simulink model "delay_on_off_prove"  (R2014b)
settings: Solver=FixedStepDiscrete  StartTime=0.0  StopTime=10.0  FixedStep=0.01  RelTol=1e-3
undefined symbols (not defined in the file): sldvsubsys
libraries: sldvlib x24
settings Model: ModifiedByFormat=Natasha  Creator=Natasha  LastModifiedBy=Natasha
settings DebuggingCC: UnderspecifiedInitializationDetection=Classic  MergeDetectMultiDrivingBlocksExec=none
settings ConfigComp: Description=Design Verifier Custom Configuration Component  DVMaxProcessTime=3600  DVMaxTestCaseSteps=500  DVTestSuiteOptimization=CombinedObjectives (Nonlinear Extended)  DVDetectActiveLogic=on

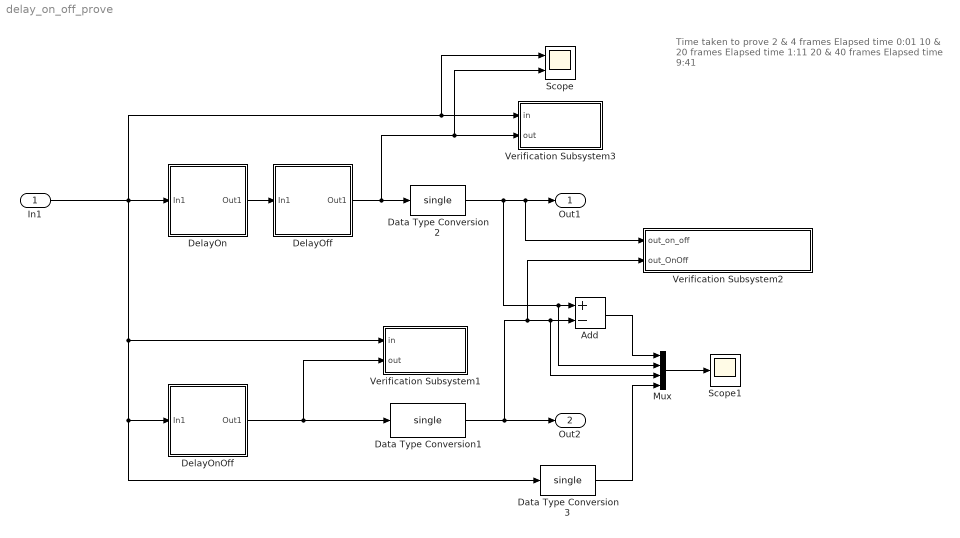
== system delay_on_off_prove ==
  note: Time taken to prove
      |
      | 2 & 4 frames Elapsed time 0:01
      | 10 & 20 frames Elapsed time 1:11
      | 20 & 40 frames Elapsed time 9:41
  In1 : Inport
  Add : Sum  Inputs=+-
  Data Type Conversion1 : DataTypeConversion  OutDataTypeStr=single
  Data Type Conversion2 : DataTypeConversion  OutDataTypeStr=single
  Data Type Conversion3 : DataTypeConversion  OutDataTypeStr=single
  DelayOff : Subsystem
  DelayOn : Subsystem
  DelayOnOff : Subsystem
  Mux : Mux
  Scope : Scope  NumInputPorts=2
      settings: YMin=-5~-5  YMax=5~5
  Scope1 : Scope
  Verification Subsystem1 : Subsystem  Tag=VerificationSubsystem  DisableCoverage=on  LoadFcn=sldvsubsys('check')  TreatAsAtomicUnit=on  SimViewingDevice=on  mask(VerificationSubsystem){}
      mask init:
      | sldvsubsys('maskInit');
      settings: CopyFcn=sldvsubsys('copy');  OpenFcn=open_system(gcb,'force');
      settings: PreSaveFcn=|
      | set_param(gcb,'SimViewingDevice','on');
      | sldvsubsys('check');
      mask Help: helpview(fullfile(docroot,'toolbox','sldv','sldv.map'),'verificationsubsystem')
      mask Display: image(imread('sldvicon_versubsys.png','BackGroundColor',[1 1 1]),'center');
  Verification Subsystem2 : Subsystem  Tag=VerificationSubsystem  DisableCoverage=on  LoadFcn=sldvsubsys('check')  TreatAsAtomicUnit=on  SimViewingDevice=on  mask(VerificationSubsystem){}
      mask init:
      | sldvsubsys('maskInit');
      settings: CopyFcn=sldvsubsys('copy');  OpenFcn=open_system(gcb,'force');
      settings: PreSaveFcn=|
      | set_param(gcb,'SimViewingDevice','on');
      | sldvsubsys('check');
      mask Help: helpview(fullfile(docroot,'toolbox','sldv','sldv.map'),'verificationsubsystem')
      mask Display: image(imread('sldvicon_versubsys.png','BackGroundColor',[1 1 1]),'center');
  Verification Subsystem3 : Subsystem  Tag=VerificationSubsystem  DisableCoverage=on  LoadFcn=sldvsubsys('check')  TreatAsAtomicUnit=on  SimViewingDevice=on  mask(VerificationSubsystem){}
      mask init:
      | sldvsubsys('maskInit');
      settings: CopyFcn=sldvsubsys('copy');  OpenFcn=open_system(gcb,'force');
      settings: PreSaveFcn=|
      | set_param(gcb,'SimViewingDevice','on');
      | sldvsubsys('check');
      mask Help: helpview(fullfile(docroot,'toolbox','sldv','sldv.map'),'verificationsubsystem')
      mask Display: image(imread('sldvicon_versubsys.png','BackGroundColor',[1 1 1]),'center');
  Out1 : Outport
  Out2 : Outport  Port=2
  wires:
  DelayOn/1(Out1) -> DelayOff/1(In1)
  DelayOff/1(Out1) -> Data Type Conversion2/1, Verification Subsystem3/2(out), Scope/2
  DelayOnOff/1(Out1) -> Verification Subsystem1/2(out), Data Type Conversion1/1
  Add/1 -> Mux/1
  Data Type Conversion1/1 -> Verification Subsystem2/2(out_OnOff), Mux/3, Add/2, Out2/1
  Data Type Conversion2/1 -> Mux/2, Add/1, Verification Subsystem2/1(out_on_off), Out1/1
  Mux/1 -> Scope1/1
  In1/1 -> Verification Subsystem3/1(in), Scope/1, Verification Subsystem1/1(in), Data Type Conversion3/1, DelayOnOff/1(In1), DelayOn/1(In1)
  Data Type Conversion3/1 -> Mux/4

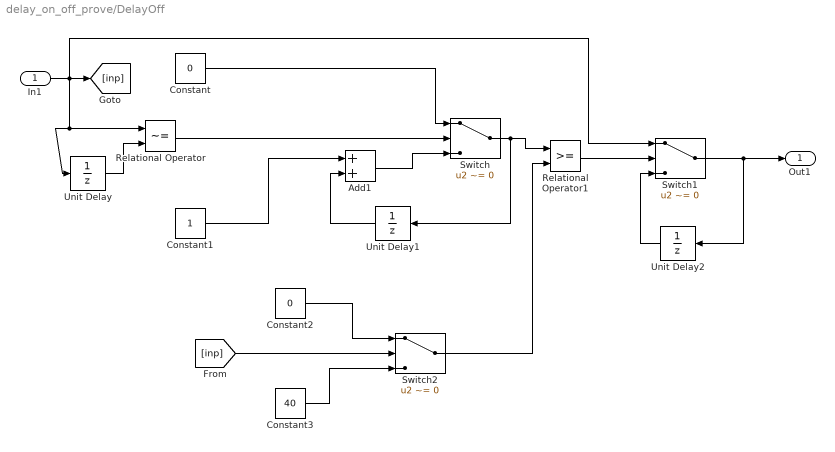
== system delay_on_off_prove/DelayOff ==
  In1 : Inport
  Add1 : Sum
  Constant : Constant  Value=0
  Constant1 : Constant
  Constant2 : Constant  Value=0
  Constant3 : Constant  Value=40
  Relational Operator : RelationalOperator  Operator=~=  OutDataTypeStr=boolean
  Relational Operator1 : RelationalOperator  OutDataTypeStr=boolean
  Switch : Switch  Criteria=u2 ~= 0
  Switch1 : Switch  Criteria=u2 ~= 0
  Switch2 : Switch  Criteria=u2 ~= 0
  Unit Delay : UnitDelay  SampleTime=-1
  Unit Delay1 : UnitDelay  SampleTime=-1
  Unit Delay2 : UnitDelay  SampleTime=-1
  Out1 : Outport
  wires:
  In1/1 -> [inp], Relational Operator/1, Unit Delay/1, Switch1/1
  [inp] -> Switch2/2
  Add1/1 -> Switch/3
  Switch2/1 -> Relational Operator1/2
  Constant3/1 -> Switch2/3
  Switch/1 -> Relational Operator1/1, Unit Delay1/1
  Relational Operator1/1 -> Switch1/2
  Unit Delay2/1 -> Switch1/3
  Switch1/1 -> Unit Delay2/1, Out1/1
  Unit Delay/1 -> Relational Operator/2
  Constant/1 -> Switch/1
  Relational Operator/1 -> Switch/2
  Constant1/1 -> Add1/1
  Constant2/1 -> Switch2/1
  Unit Delay1/1 -> Add1/2

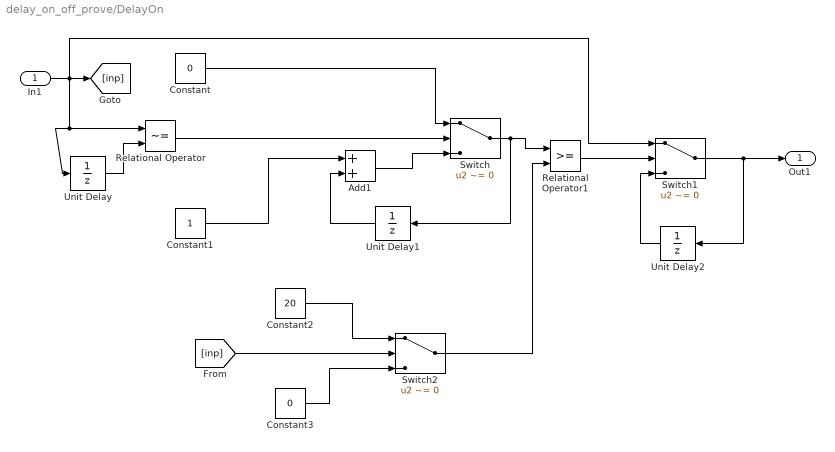
== system delay_on_off_prove/DelayOn ==
  In1 : Inport
  Add1 : Sum
  Constant : Constant  Value=0
  Constant1 : Constant
  Constant2 : Constant  Value=20
  Constant3 : Constant  Value=0
  Relational Operator : RelationalOperator  Operator=~=  OutDataTypeStr=boolean
  Relational Operator1 : RelationalOperator  OutDataTypeStr=boolean
  Switch : Switch  Criteria=u2 ~= 0
  Switch1 : Switch  Criteria=u2 ~= 0
  Switch2 : Switch  Criteria=u2 ~= 0
  Unit Delay : UnitDelay  SampleTime=-1
  Unit Delay1 : UnitDelay  SampleTime=-1
  Unit Delay2 : UnitDelay  SampleTime=-1
  Out1 : Outport
  wires:
  Unit Delay1/1 -> Add1/2
  Constant2/1 -> Switch2/1
  Constant1/1 -> Add1/1
  Relational Operator/1 -> Switch/2
  Constant/1 -> Switch/1
  Unit Delay/1 -> Relational Operator/2
  Switch1/1 -> Out1/1, Unit Delay2/1
  Unit Delay2/1 -> Switch1/3
  Relational Operator1/1 -> Switch1/2
  Switch/1 -> Unit Delay1/1, Relational Operator1/1
  Constant3/1 -> Switch2/3
  Switch2/1 -> Relational Operator1/2
  Add1/1 -> Switch/3
  [inp] -> Switch2/2
  In1/1 -> Switch1/1, Unit Delay/1, Relational Operator/1, [inp]

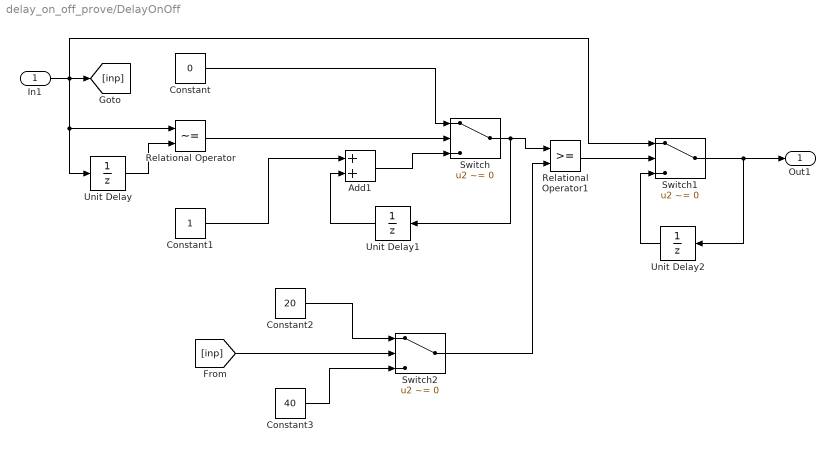
== system delay_on_off_prove/DelayOnOff ==
  In1 : Inport
  Add1 : Sum
  Constant : Constant  Value=0
  Constant1 : Constant
  Constant2 : Constant  Value=20
  Constant3 : Constant  Value=40
  Relational Operator : RelationalOperator  Operator=~=  OutDataTypeStr=boolean
  Relational Operator1 : RelationalOperator  OutDataTypeStr=boolean
  Switch : Switch  Criteria=u2 ~= 0
  Switch1 : Switch  Criteria=u2 ~= 0
  Switch2 : Switch  Criteria=u2 ~= 0
  Unit Delay : UnitDelay  SampleTime=-1
  Unit Delay1 : UnitDelay  SampleTime=-1
  Unit Delay2 : UnitDelay  SampleTime=-1
  Out1 : Outport
  wires:
  Unit Delay1/1 -> Add1/2
  Constant2/1 -> Switch2/1
  Constant1/1 -> Add1/1
  Relational Operator/1 -> Switch/2
  Constant/1 -> Switch/1
  Unit Delay/1 -> Relational Operator/2
  Switch1/1 -> Out1/1, Unit Delay2/1
  Unit Delay2/1 -> Switch1/3
  Relational Operator1/1 -> Switch1/2
  Switch/1 -> Unit Delay1/1, Relational Operator1/1
  Constant3/1 -> Switch2/3
  Switch2/1 -> Relational Operator1/2
  Add1/1 -> Switch/3
  [inp] -> Switch2/2
  In1/1 -> Switch1/1, Unit Delay/1, Relational Operator/1, [inp]

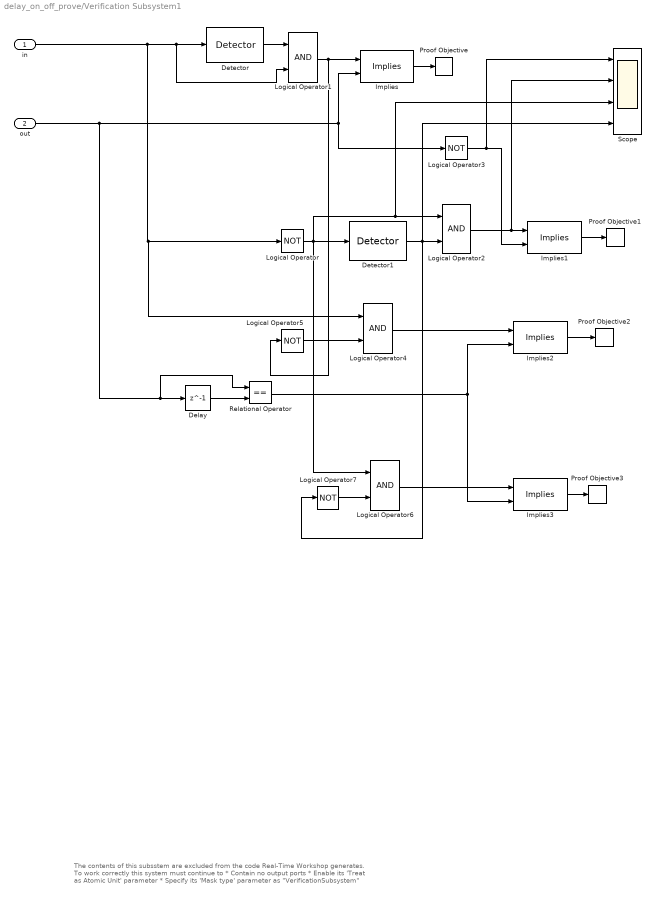
== system delay_on_off_prove/Verification Subsystem1 ==
  note: The contents of this subsstem are excluded from the code Real-Time
      | Workshop generates.
      |
      | To work correctly this system must continue to
      | * Contain no output ports
      | * Enable its 'Treat as Atomic Unit' parameter
      | * Specify its 'Mask type' parameter as "VerificationSubsystem"
  in : Inport
  out : Inport  Port=2
  Delay : Delay  DelayLength=1  InitialCondition=0
  Detector : sldvlib/Temporal Operators/Detector  reset=off  typ=Synchronized  in_hold=21  delay=1  out_hold=3
  Detector1 : sldvlib/Temporal Operators/Detector  reset=off  typ=Synchronized  in_hold=41  delay=1  out_hold=3
  Implies{,1..3} (4 alike) : sldvlib/Verification Utilities/Implies
  Logical Operator{,3,5,7} (4 alike) : Logic  Operator=NOT  AllPortsSameDT=off  OutDataTypeStr=boolean
  Logical Operator{1..2,4,6} (4 alike) : Logic  AllPortsSameDT=off  OutDataTypeStr=boolean
  Proof Objective{,1..3} (4 alike) : sldvlib/Objectives and Constraints/Proof Objective  enabled=on  customAVTBlockType=Proof Objective  intervals=true  dispValues=on  outEnabled=off  enableStopSim=on
      settings: AttributesFormatString=%<intervals>
  Relational Operator : RelationalOperator  Operator===  OutDataTypeStr=boolean
  Scope : Scope  NumInputPorts=4
      settings: YMin=-5~-5~-5~-5  YMax=5~5~5~5  SaveName=ScopeData2
  wires:
  Implies3/1 -> Proof Objective3/1
  Logical Operator6/1 -> Implies3/1
  Detector1/1 -> Logical Operator2/2, Scope/4, Logical Operator7/1
  Logical Operator7/1 -> Logical Operator6/2
  Logical Operator1/1 -> Implies/1, Logical Operator5/1
  Implies2/1 -> Proof Objective2/1
  Relational Operator/1 -> Implies3/2, Implies2/2
  Logical Operator4/1 -> Implies2/1
  Logical Operator5/1 -> Logical Operator4/2
  out/1 -> Implies/2, Logical Operator3/1, Delay/1, Relational Operator/1
  Delay/1 -> Relational Operator/2
  Implies1/1 -> Proof Objective1/1
  Logical Operator3/1 -> Implies1/2, Scope/1
  Logical Operator2/1 -> Implies1/1, Scope/2
  Logical Operator/1 -> Detector1/1, Logical Operator2/1, Scope/3, Logical Operator6/1
  in/1 -> Detector/1, Logical Operator1/2, Logical Operator/1, Logical Operator4/1
  Implies/1 -> Proof Objective/1
  Detector/1 -> Logical Operator1/1

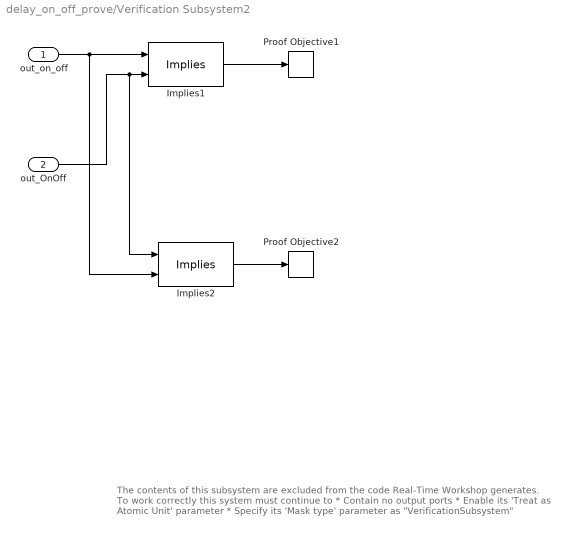
== system delay_on_off_prove/Verification Subsystem2 ==
  note: The contents of this subsystem are excluded from the code Real-Time
      | Workshop generates.
      |
      | To work correctly this system must continue to
      | * Contain no output ports
      | * Enable its 'Treat as Atomic Unit' parameter
      | * Specify its 'Mask type' parameter as "VerificationSubsystem"
  out_on_off : Inport
  out_OnOff : Inport  Port=2
  Implies1 : sldvlib/Verification Utilities/Implies
  Implies2 : sldvlib/Verification Utilities/Implies
  Proof Objective1 : sldvlib/Objectives and Constraints/Proof Objective  enabled=on  customAVTBlockType=Proof Objective  intervals=true  dispValues=on  outEnabled=off  enableStopSim=on
      settings: AttributesFormatString=%<intervals>
  Proof Objective2 : sldvlib/Objectives and Constraints/Proof Objective  enabled=on  customAVTBlockType=Proof Objective  intervals=true  dispValues=on  outEnabled=off  enableStopSim=on
      settings: AttributesFormatString=%<intervals>
  wires:
  out_on_off/1 -> Implies2/2, Implies1/1
  out_OnOff/1 -> Implies2/1, Implies1/2
  Implies1/1 -> Proof Objective1/1
  Implies2/1 -> Proof Objective2/1

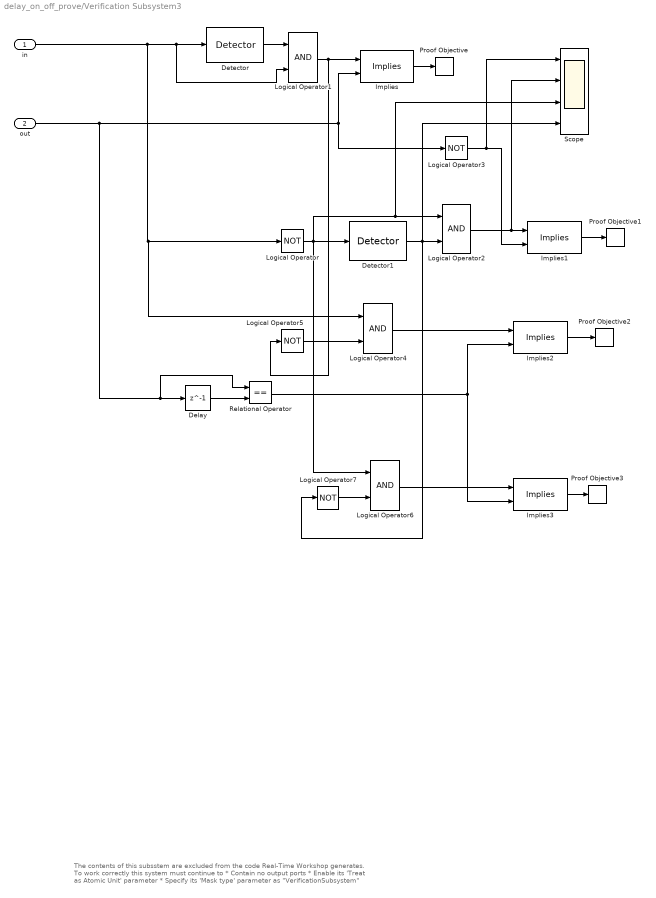
== system delay_on_off_prove/Verification Subsystem3 ==
  note: The contents of this subsstem are excluded from the code Real-Time
      | Workshop generates.
      |
      | To work correctly this system must continue to
      | * Contain no output ports
      | * Enable its 'Treat as Atomic Unit' parameter
      | * Specify its 'Mask type' parameter as "VerificationSubsystem"
  in : Inport
  out : Inport  Port=2
  Delay : Delay  DelayLength=1  InitialCondition=0
  Detector : sldvlib/Temporal Operators/Detector  reset=off  typ=Synchronized  in_hold=21  delay=1  out_hold=3
  Detector1 : sldvlib/Temporal Operators/Detector  reset=off  typ=Synchronized  in_hold=41  delay=1  out_hold=3
  Implies{,1..3} (4 alike) : sldvlib/Verification Utilities/Implies
  Logical Operator{,3,5,7} (4 alike) : Logic  Operator=NOT  AllPortsSameDT=off  OutDataTypeStr=boolean
  Logical Operator{1..2,4,6} (4 alike) : Logic  AllPortsSameDT=off  OutDataTypeStr=boolean
  Proof Objective{,1..3} (4 alike) : sldvlib/Objectives and Constraints/Proof Objective  enabled=on  customAVTBlockType=Proof Objective  intervals=true  dispValues=on  outEnabled=off  enableStopSim=on
      settings: AttributesFormatString=%<intervals>
  Relational Operator : RelationalOperator  Operator===  OutDataTypeStr=boolean
  Scope : Scope  NumInputPorts=4
      settings: YMin=-5~-5~-5~-5  YMax=5~5~5~5  SaveName=ScopeData2
  wires:
  Detector/1 -> Logical Operator1/1
  Implies/1 -> Proof Objective/1
  in/1 -> Logical Operator4/1, Logical Operator/1, Logical Operator1/2, Detector/1
  Logical Operator/1 -> Logical Operator6/1, Scope/3, Logical Operator2/1, Detector1/1
  Logical Operator2/1 -> Scope/2, Implies1/1
  Logical Operator3/1 -> Scope/1, Implies1/2
  Implies1/1 -> Proof Objective1/1
  Delay/1 -> Relational Operator/2
  out/1 -> Relational Operator/1, Delay/1, Logical Operator3/1, Implies/2
  Logical Operator5/1 -> Logical Operator4/2
  Logical Operator4/1 -> Implies2/1
  Relational Operator/1 -> Implies2/2, Implies3/2
  Implies2/1 -> Proof Objective2/1
  Logical Operator1/1 -> Logical Operator5/1, Implies/1
  Logical Operator7/1 -> Logical Operator6/2
  Detector1/1 -> Logical Operator7/1, Scope/4, Logical Operator2/2
  Logical Operator6/1 -> Implies3/1
  Implies3/1 -> Proof Objective3/1
